simulink model "model_inner"  (R2015a)
settings: Solver=ode45  StartTime=0.0  StopTime=Tfin  RelTol=1e-3
values from neighbouring files (symbols this model uses):
  init_in = [0;0]    [main_parts.m]
  init_in_dot = [0;0]    [main_parts.m]
undefined symbols (not defined in the file or in its folder): K, param
settings Model: Creator=jesus  LastModifiedBy=jesus

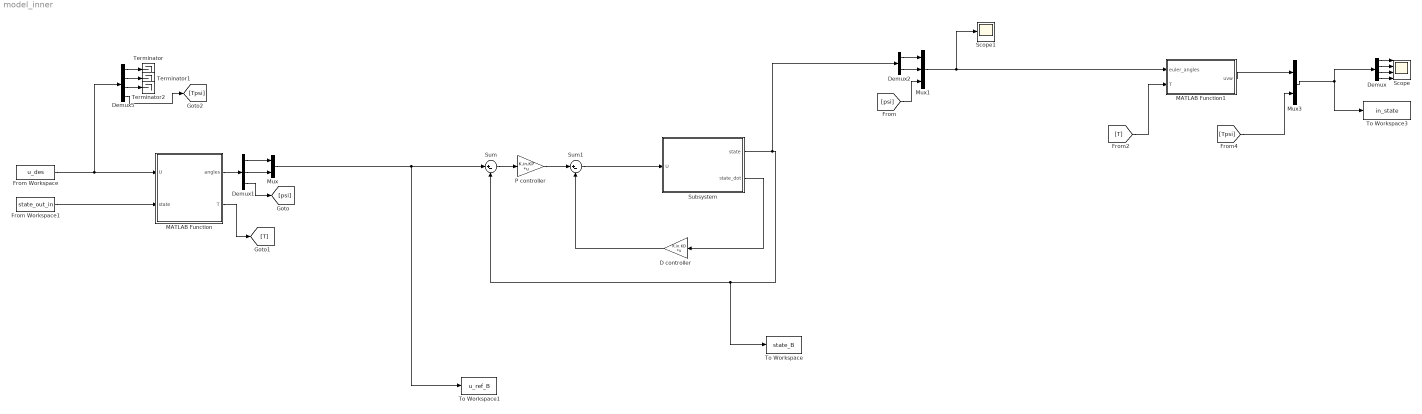
== system model_inner ==
  D controller : Gain  Gain=K.in.KD  Multiplication=Matrix(K*u)
  Demux : Demux
  Demux1 : Demux  Outputs=3
  Demux2 : Demux  Outputs=2
  Demux5 : Demux
  From Workspace : FromWorkspace  VariableName=u_des  SampleTime=param.hs  Interpolate=off  OutputAfterFinalValue=Setting to zero
  From Workspace1 : FromWorkspace  VariableName=state_out_in  SampleTime=param.hs  Interpolate=off  OutputAfterFinalValue=Setting to zero
  MATLAB Function : MATLAB Function  TreatAsAtomicUnit=on
  MATLAB Function1 : MATLAB Function  TreatAsAtomicUnit=on
  Mux : Mux  Inputs=2
  Mux1 : Mux  Inputs=3
  Mux3 : Mux  Inputs=2
  P controller : Gain  Gain=K.in.KP  Multiplication=Matrix(K*u)
  Scope : Scope  NumInputPorts=4
      settings: YMin=-5~-5~-5~-5  YMax=5~5~5~5
  Scope1 : Scope
  Subsystem : Subsystem
  Sum : Sum  Inputs=|+-
  Sum1 : Sum  Inputs=|+-
  Terminator : Terminator
  Terminator1 : Terminator
  Terminator2 : Terminator
  To Workspace : ToWorkspace  VariableName=state_B  SaveFormat=Structure With Time  SampleTime=-1
  To Workspace1 : ToWorkspace  VariableName=u_ref_B  SaveFormat=Structure With Time  SampleTime=-1
  To Workspace3 : ToWorkspace  VariableName=in_state  SaveFormat=Structure With Time  SampleTime=-1
  wires:
  From Workspace/1 -> Demux5/1, MATLAB Function/1(U)
  Sum1/1 -> Subsystem/1(U)
  Sum/1 -> P controller/1
  P controller/1 -> Sum1/1
  D controller/1 -> Sum1/2
  Subsystem/2(state_dot) -> D controller/1
  Subsystem/1(state) -> Demux2/1, To Workspace/1, Sum/2
  Demux/1 -> Scope/1
  Demux/2 -> Scope/2
  Demux/3 -> Scope/3
  Demux/4 -> Scope/4
  Mux/1 -> To Workspace1/1, Sum/1
  From Workspace1/1 -> MATLAB Function/2(state)
  Demux1/1 -> Mux/1
  Demux1/2 -> Mux/2
  MATLAB Function/1(angles) -> Demux1/1
  Demux1/3 -> [psi]
  Demux2/2 -> Mux1/2
  Demux2/1 -> Mux1/1
  Mux1/1 -> MATLAB Function1/1(euler_angles), Scope1/1
  [psi] -> Mux1/3
  MATLAB Function/2(T) -> [T]
  [T] -> MATLAB Function1/2(T)
  Demux5/4 -> [Tpsi]
  Demux5/1 -> Terminator/1
  Demux5/2 -> Terminator1/1
  Demux5/3 -> Terminator2/1
  [Tpsi] -> Mux3/2
  Mux3/1 -> To Workspace3/1, Demux/1
  MATLAB Function1/1(uvw) -> Mux3/1

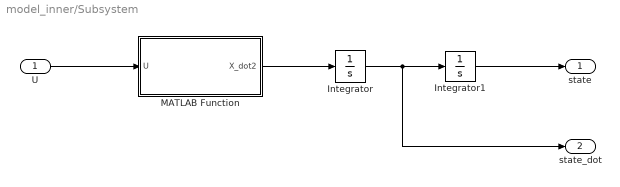
== system model_inner/Subsystem ==
  U : Inport
  Integrator : Integrator  InitialCondition=init_in_dot
  Integrator1 : Integrator  InitialCondition=init_in
  MATLAB Function : MATLAB Function  TreatAsAtomicUnit=on
  state : Outport
  state_dot : Outport  Port=2
  wires:
  Integrator/1 -> state_dot/1, Integrator1/1
  Integrator1/1 -> state/1
  U/1 -> MATLAB Function/1(U)
  MATLAB Function/1(X_dot2) -> Integrator/1

== matlab function model_inner/MATLAB Function ==
  data: U input; angles output; state input; T output
function [angles, T] = fcn1(U, state)
%#codegen
% Mathematical derivation of formulas in XXXX

% Inputs
    u_abs = U(1);   v_abs = U(2);   w_abs = U(3);
    Tpsi = U(4);
    psi = state(4);
    
% Torque
T = sqrt( u_abs^2 + v_abs^2 + w_abs^2 );

% normalization of thrust components
u = u_abs/T;
v = v_abs/T;
w = w_abs/T;

% Euler angles

    % Considering w =! 0 (always true)
    %   Considering phi and theta are never 90º (iff w=!0)    

     % psi is a known value
        a = cos(psi);
        b = sin(psi);

    % compute phi & theta
    if ( u ~= 0 && v ~=0 )
        if ( a==0 )
            phi   = asinn( u/b );
            theta = atann( v/(w*b) );   
        elseif ( b==0 )
            phi   = asinn( -v/a );
            theta = atann( u/(w*a) );
        else
            aux = (u-v*w) / (b*(1+w));
            phi   = asinn( aux );
            theta = atann ( (u-b*aux) / (w*a) );
        end

    elseif ( u == 0 && v == 0 )
        phi   = 0;
        theta = 0;

    elseif ( u == 0 && v ~= 0 )
        if ( a==0 )
            phi   = 0;
            theta = atann ( v/(b*w) );
        elseif ( b==0 )
            phi   = asinn( -v/a );
            theta = 0;
        else
            phi   = asinn( -a*v );
            theta = atann( b*v/w );
        end

    elseif ( u ~=0 && v == 0 )
        if ( a==0 )
            phi   = asinn( b*u );
            theta = 0;
        elseif ( b==0 )
            phi   = 0;
            theta = atann( u/(a*w) );
        else 
            phi   = asinn( b*u );
            theta = atann( a*u/w);
        end
    else
        phi = pi/3;
        theta = pi/3;
    end
        angles = [phi, theta, psi]';
end


function [ angle ] = asinn( aa )
    angle = asin(aa);
    % angle correction
    if ~( -pi/2 < angle < pi/2 )
        angle = angle - pi/2;
    end
end

function [ angle ] = atann( aa )
    angle = atan(aa);
    % angle correction
    if ~( -pi/2 < angle < pi/2 )
        angle = angle - pi/2;
    end
end

== matlab function model_inner/MATLAB Function1 ==
  data: euler_angles input; uvw output; T input
function uvw  = fcn2( euler_angles, T )
%#codegen
% call RT2uvw

% inputs
    phi   = euler_angles(1);
    theta = euler_angles(2);
    Psi   = euler_angles(3);
    
% rotation matrix
    R = [cos(theta)*cos(Psi)  sin(phi)*sin(theta)*cos(Psi)-cos(phi)*sin(Psi)  cos(phi)*sin(theta)*cos(Psi)+sin(phi)*sin(Psi)
         cos(theta)*sin(Psi)  sin(phi)*sin(theta)*sin(Psi)+cos(phi)*sin(Psi)  cos(phi)*sin(theta)*sin(Psi)-sin(phi)*cos(Psi)
         -sin(theta)          sin(phi)*cos(theta)                             cos(phi)*cos(theta)                           ];

    
    
%     uvw = eul2rotm( euler_angles' ) * [0;0;T];
%uvw = [];
uvw = R* [0;0;T];

== matlab function model_inner/Subsystem/MATLAB Function ==
  data: U input; X_dot2 output
function X_dot2   = sys_in ( U )
%#codegen
% parameters
    Ix = 0.002237568100000;   
    Iy = 0.002985236000000;

X_dot2 = [ 0; 0];
X_dot2(1) = U(1) / Iy;
X_dot2(2) = U(2) / Ix;
